simulink model "RESONANT_LOAD"  (R2024b)
settings: Solver=VariableStepAuto  StartTime=0.0  StopTime=10.0  RelTol=1e-3
undefined symbols (not defined in the file or in its folder): denBeam, kappa, numBeam
settings Model: Creator=llp  LastModifiedBy=llp

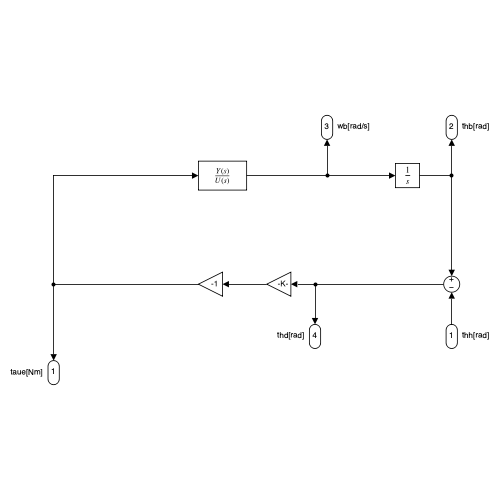
[thumbnail: Simulink's stored preview of the top-level diagram]
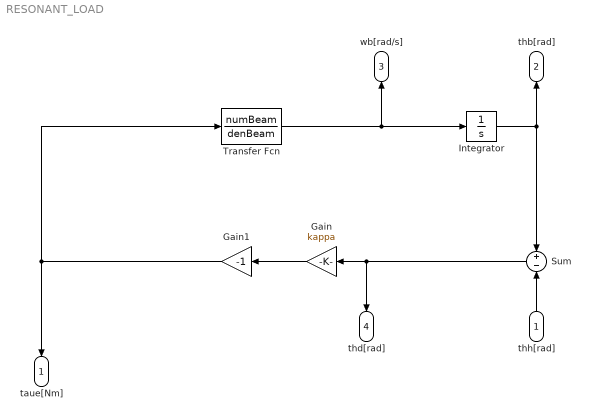
== system RESONANT_LOAD ==
  thh[rad] : Inport
  Gain : Gain  Gain=kappa
  Gain1 : Gain  Gain=-1
  Integrator : Integrator
  Sum : Sum  Inputs=+-
  Transfer Fcn : TransferFcn  Numerator=numBeam  Denominator=denBeam
  taue[Nm] : Outport
  thb[rad] : Outport  Port=2
  wb[rad/s] : Outport  Port=3
  thd[rad] : Outport  Port=4
  wires:
  Integrator/1 -> Sum/1, thb[rad]/1
  thh[rad]/1 -> Sum/2
  Sum/1 -> Gain/1, thd[rad]/1
  Gain/1 -> Gain1/1
  Transfer Fcn/1 -> Integrator/1, wb[rad/s]/1
  Gain1/1 -> taue[Nm]/1, Transfer Fcn/1
